simulink model "transition_RLSMC_2024aR1"  (R2024a)
settings: Solver=ode4  StartTime=0.0  StopTime=55  FixedStep=0.002  RelTol=1e-3
InitFcn:
  | model_init_param
values from neighbouring files (symbols this model uses):
  ModelInit_AngEuler = [ModelInit_phi, ModelInit_theta, ModelInit_psi]    [model_init_param.m]
  ModelInit_g = 9.80665    [model_init_param.m]
  ModelInit_PosE = [ModelInit_PosX, ModelInit_PosY, ModelInit_PosZ]    [model_init_param.m]
  ModelInit_RateB = [0, 0, 0]    [model_init_param.m]
  ModelInit_trim_da = 0    [model_init_param.m]
  ModelInit_trim_de = 0    [model_init_param.m]
  ModelInit_trim_dr = 0    [model_init_param.m]
  ModelInit_trim_dT = 0    [model_init_param.m]
  ModelInit_trim_u = ModelParam_mass/(4*ModelParam_rotor_Kf)    (= 0.533231666667)    [model_init_param.m]
  ModelInit_VelB = [ModelInit_Velx, ModelInit_Vely, ModelInit_Velz]    [model_init_param.m]
  ModelParam_Ixx = 2.957616474    [model_init_param.m]
  ModelParam_Iyy = 5.552907742    [model_init_param.m]
  ModelParam_Izz = 8.264706552    [model_init_param.m]
  ModelParam_mass = 31.9939    [model_init_param.m]
  ModelParam_rotor_Kf = 15    [model_init_param.m]
  ModelParam_rotor_Kt = 2.45    [model_init_param.m]
  ModelParam_rotor_x = 1.25    [model_init_param.m]
  ModelParam_rotor_y = 1.3    [model_init_param.m]
undefined symbols (not defined in the file or in its folder): Newton, Raphson, sigbuilder_block
libraries: aerolibconvert2 x5, aerolibasang x5, sharedutil x2, simulink x2, sharedtransform x2, aerolibatmos2 x1
settings Model: Creator=yifangfu  LastModifiedBy=yifangfu

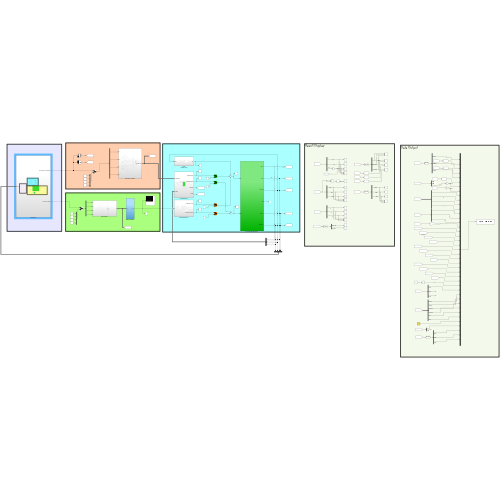
[thumbnail: Simulink's stored preview of the top-level diagram]
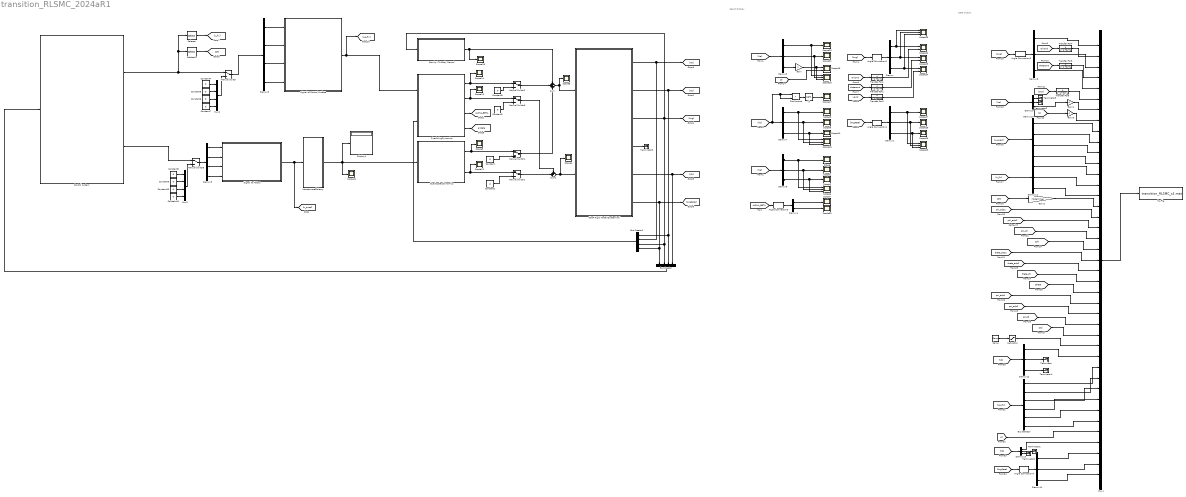
== system transition_RLSMC_2024aR1 ==
  note: Result Display
  note: Data Output
  6DoF Rigid Model(Quaternion) : Subsystem
  Actuator coefficiency : Subsystem
  Angle Conversion{1..5} (5 alike) : aerolibconvert2/Angle Conversion  IU=rad  OU=deg
  Bus Creator : BusCreator  Inputs=4
  Bus Creator1 : BusCreator  Inputs=4
  Bus Selector : BusSelector  OutputSignals=deup1,deup2,dedown1,dedown2,da1,da2
  Constant{,1..11} (12 alike) : Constant  Value=0
  Control system : Subsystem
  Demux{,1..2,6..9,11..14} (11 alike) : Demux  Outputs=3
  Demux10 : Demux
  Demux3 : Demux
  Demux4 : Demux  Outputs=2
  Demux5 : Demux
  Display4 : Display
  Dot Product : DotProduct  OutDataTypeStr=Inherit: Inherit via internal rule
  FixedWingDynamics : Subsystem
  Gain : Gain
  Gain1 : Gain  Gain=-1
  Gain2 : Gain  Gain=ModelInit_g
  Gain3 : Gain  Gain=-1
  Gravity (To Body Frame) : Subsystem
  Manual Switch{,1..2,4..6} (6 alike) : ManualSwitch
  Mux2 : Mux
  Mux3 : Mux
  Mux4 : Mux  Inputs=41
  QuadcoptersDynamics : Subsystem
  Ramp : simulink/Sources/Ramp  slope=0.65  start=0  InitialOutput=5
  Saturation : Saturate  UpperLimit=25
  Scope{,1..5,7..15,17,20..21,26..28,30} (22 alike) : Scope
  Scope{6,16,19,25,29} (5 alike) : Scope  NumInputPorts=3
  Scope{18,22..24} (4 alike) : Scope  NumInputPorts=2
  Selector : Selector  InputPortWidth=4  IndexOptions=Index vector (dialog)  Indices=[1 2 3]  OutputSizes=1
  Selector1 : Selector  InputPortWidth=4  IndexOptions=Index vector (dialog)  Indices=[4]  OutputSizes=1
  Signal to Control Surface : Subsystem
  Signal to Motors : Subsystem
  Sum : Sum  Inputs=+++
  Sum1 : Sum  Inputs=++|
  Terminator{,1..6} (7 alike) : Terminator
  To File : ToFile  Filename=transition_RLSMC_s1.mat  MatrixName=RLSMC_s1
  Transfer Fcn{1..6} (6 alike) : TransferFcn  Numerator=[4]  Denominator=[1 3 4]
  vt : Math  Operator=sqrt  SignedPower=on
  tag scope: ALPHA_BETA=global, airdata=global
  wires:
  Gain/1 -> Scope19/3, Scope18/1  "Height_m"
  Demux2/3 -> Gain/1  "Z_m"
  [yawd] -> Transfer Fcn3/1
  [Xe] -> Demux2/1
  Demux6/2 -> Scope6/2, Scope1/1  "vy"
  [ALPHA_BETA] -> Angle Conversion3/1
  [thetacmd] -> Transfer Fcn2/1
  Demux6/3 -> Scope6/3, Scope2/1  "vz"
  Demux7/3 -> Scope16/3, Scope10/1  "w(m/s)"
  Transfer Fcn3/1 -> Scope24/2
  Demux2/2 -> Scope19/2, Scope21/1  "Y_m"
  Dot Product/1 -> vt/1
  Demux2/1 -> Scope19/1, Scope20/1  "X_m"
  Demux/1 -> Scope22/1, Scope25/1  "phi(deg)"
  Demux4/1 -> Scope7/1  "alpha_deg"
  Demux/3 -> Scope24/1, Scope25/3  "psi(deg)"
  Demux1/3 -> Scope26/1, Scope29/3  "r(deg)"
  Demux1/1 -> Scope27/1, Scope29/1  "p(deg)"
  [Ve] -> Demux6/1
  [rollcmd] -> Transfer Fcn1/1
  Demux6/1 -> Scope6/1, Scope/1  "vx"
  Transfer Fcn2/1 -> Scope23/2
  [zd] -> Scope18/2
  [Ang] -> Angle Conversion2/1
  Angle Conversion1/1 -> Demux1/1
  Demux4/2 -> Scope30/1  "beta_deg"
  [Vb] -> Dot Product/2, Dot Product/1, Demux7/1
  Transfer Fcn1/1 -> Scope22/2
  [AngRate] -> Angle Conversion1/1
  Demux/2 -> Scope23/1, Scope25/2  "theta(deg)"
  Demux7/1 -> Scope16/1, Scope8/1  "u(m/s)"
  Angle Conversion3/1 -> Demux4/1
  vt/1 -> Scope17/1  "V(m/s)"
  Demux1/2 -> Scope28/1, Scope29/2  "q(deg)"
  Demux7/2 -> Scope16/2, Scope9/1  "v(m/s)"
  Angle Conversion2/1 -> Demux/1
  6DoF Rigid Model(Quaternion)/5("vb(m/s) ") -> [Vb], Bus Creator/4  "uvw"
  6DoF Rigid Model(Quaternion)/4(Rbe) -> Terminator3/1
  6DoF Rigid Model(Quaternion)/1(ve(m/s)) -> [Ve], Bus Creator1/2  "Ve"
  6DoF Rigid Model(Quaternion)/6("p,q,r(rad/s) ") -> Bus Creator1/4, Bus Creator/1, [AngRate]  "pqr"
  6DoF Rigid Model(Quaternion)/2("xe(m) ") -> [Xe], Bus Creator1/1, Bus Creator/3  "Xe"
  6DoF Rigid Model(Quaternion)/3(Euler(rad)) -> Gravity (To Body Frame)/1(Euler), [Ang], Bus Creator1/3, Bus Creator/2  "euler"
  Demux5/2 -> Signal to Motors/2(u2)
  Demux5/1 -> Signal to Motors/1(u1)
  Actuator coefficiency/1(u_out) -> QuadcoptersDynamics/1(u), Scope11/1, Display4/1
  Demux5/4 -> Signal to Motors/4(u4)
  Signal to Motors/1(u) -> [u_quad], Actuator coefficiency/1(u_in)
  Demux5/3 -> Signal to Motors/3(u3)
  Constant9/1 -> Mux3/2
  Constant10/1 -> Mux3/3
  Constant11/1 -> Mux3/4
  Mux3/1 -> Manual Switch5/2
  Constant8/1 -> Mux3/1
  Manual Switch5/1 -> Demux5/1
  Control system/2(ControlInputs_Rotors) -> Manual Switch5/1
  Bus Creator/1 -> Control system/1(Uav State)
  Sum/1 -> 6DoF Rigid Model(Quaternion)/1(fb), Scope3/1
  Gravity (To Body Frame)/1(g_b) -> Scope15/1, Sum/1
  FixedWingDynamics/3(alpha beta) -> [ALPHA_BETA]
  FixedWingDynamics/4(Airdata) -> [airdata]
  QuadcoptersDynamics/1(Quadcopters Force) -> Manual Switch4/1, Scope5/1
  FixedWingDynamics/1(FixedWing Force) -> Scope14/1, Manual Switch2/1
  Sum1/1 -> 6DoF Rigid Model(Quaternion)/2(Mb), Scope4/1
  QuadcoptersDynamics/2(Quadcopters Moment) -> Manual Switch1/1, Scope12/1
  FixedWingDynamics/2(FixedWing Moment) -> Manual Switch6/1, Scope13/1
  Constant/1 -> Manual Switch4/2
  Constant1/1 -> Manual Switch1/2
  Manual Switch1/1 -> Sum1/2
  Manual Switch4/1 -> Sum/3
  Constant2/1 -> Manual Switch6/2
  Manual Switch6/1 -> Sum1/1
  Manual Switch2/1 -> Sum/2
  Constant3/1 -> Manual Switch2/2
  Bus Creator1/1 -> FixedWingDynamics/2(UavState)
  Signal to Control Surface/1(ControlSurface) -> [ua_fix], FixedWingDynamics/1(ControlSurface)
  Constant4/1 -> Mux2/1
  Constant7/1 -> Mux2/4
  Mux2/1 -> Manual Switch/2
  Constant5/1 -> Mux2/2
  Manual Switch/1 -> Demux3/1
  Constant6/1 -> Mux2/3
  Demux3/1 -> Signal to Control Surface/1(de)
  Demux3/2 -> Signal to Control Surface/2(da)
  Demux3/3 -> Signal to Control Surface/3(dr)
  Demux3/4 -> Signal to Control Surface/4(dT)
  Control system/1(ControlInputs_ControlSurfaces) -> Selector1/1, Selector/1, Manual Switch/1
  [stheta] -> Mux4/24
  Demux11/2 -> Mux4/14  "de"
  [phi_adp2] -> Mux4/18
  Demux12/1 -> Mux4/30  "u(m/s)"
  [zd] -> Gain3/1
  [phi_adp1] -> Mux4/17
  Demux10/3 -> Mux4/11  "u3"
  Demux11/1 -> Mux4/13  "da"
  Gain2/1 -> Mux4/16
  [Xe] -> Demux9/1
  Transfer Fcn4/1 -> Mux4/2
  [dT] -> Gain2/1
  Demux9/2 -> Terminator6/1  "Y_m"
  Demux9/3 -> Gain1/1  "Z_m"
  Ramp/1 -> Saturation/1
  Transfer Fcn6/1 -> Mux4/6
  Demux8/3 -> Mux4/5  "psi(deg)"
  [Ang] -> Angle Conversion5/1
  Demux8/2 -> Mux4/3  "theta(deg)"
  Angle Conversion5/1 -> Demux8/1
  [rollcmd] -> Transfer Fcn4/1
  Gain1/1 -> Mux4/7  "Height_m"
  Demux12/3 -> Terminator4/1  "w(m/s)"
  Demux12/2 -> Terminator/1  "v(m/s)"
  [spsi] -> Mux4/28
  [psi_adp1] -> Mux4/25
  [psi_adp2] -> Mux4/26
  Demux9/1 -> Terminator5/1  "X_m"
  [phi_k3] -> Mux4/19
  Demux10/2 -> Mux4/10  "u2"
  [Vb] -> Demux12/1
  Saturation/1 -> Mux4/29  "ud"
  Demux10/4 -> Mux4/12  "u4"
  Demux10/1 -> Mux4/9  "u1"
  [psi_k3] -> Mux4/27
  Transfer Fcn5/1 -> Mux4/4
  Demux11/3 -> Mux4/15  "dr"
  [u_quad] -> Demux10/1
  Demux8/1 -> Mux4/1  "phi(deg)"
  [u_fix] -> Demux11/1
  [theta_adp2] -> Mux4/22
  [theta_k3] -> Mux4/23
  [yawd] -> Transfer Fcn6/1
  [theta_adp1] -> Mux4/21
  [thetacmd] -> Transfer Fcn5/1
  [sphi] -> Mux4/20
  Selector/1 -> [u_fix]
  Selector1/1 -> [dT]
  Mux4/1 -> To File/1
  Gain3/1 -> Mux4/8  "Height_m"
  Bus Selector/2 -> Mux4/32  "<deup2>"
  Bus Selector/1 -> Mux4/31  "<deup1>"
  Bus Selector/6 -> Mux4/36  "<da2>"
  Bus Selector/5 -> Mux4/35  "<da1>"
  Bus Selector/4 -> Mux4/34  "<dedown2>"
  Bus Selector/3 -> Mux4/33  "<dedown1>"
  [ua_fix] -> Bus Selector/1
  Demux13/1 -> Mux4/38
  Demux13/3 -> Terminator2/1
  [ud] -> Mux4/37
  [Vb] -> Demux13/1
  Demux13/2 -> Terminator1/1
  Angle Conversion4/1 -> Demux14/1
  [AngRate] -> Angle Conversion4/1
  Demux14/1 -> Mux4/39  "p(deg)"
  Demux14/2 -> Mux4/40  "q(deg)"
  Demux14/3 -> Mux4/41  "r(deg)"

== system transition_RLSMC_2024aR1/6DoF Rigid Model(Quaternion) ==
  fb : Inport
  Mb : Inport  Port=2
  Rigid-Body Dynamic Model : Subsystem
  "Rigid-Body Kinematic Model " : Subsystem
  ve(m/s) : Outport  VectorParamsAs1DForOutWhenUnconnected=off
  "xe(m) " : Outport  Port=2  VectorParamsAs1DForOutWhenUnconnected=off
  Euler(rad) : Outport  Port=3  VectorParamsAs1DForOutWhenUnconnected=off
  Rbe : Outport  Port=4  VectorParamsAs1DForOutWhenUnconnected=off
  "vb(m/s) " : Outport  Port=5  VectorParamsAs1DForOutWhenUnconnected=off
  "p,q,r(rad/s) " : Outport  Port=6  VectorParamsAs1DForOutWhenUnconnected=off
  wires:
  Rigid-Body Dynamic Model/1("p,q,r ") -> "p,q,r(rad/s) "/1, "Rigid-Body Kinematic Model "/1(pqr)
  "Rigid-Body Kinematic Model "/1(Euler) -> Euler(rad)/1
  "Rigid-Body Kinematic Model "/3(Rbe) -> Rbe/1, Rigid-Body Dynamic Model/3(Rbe)
  Mb/1 -> Rigid-Body Dynamic Model/1(Mb)
  fb/1 -> Rigid-Body Dynamic Model/2(f)
  Rigid-Body Dynamic Model/2(ve) -> ve(m/s)/1, "Rigid-Body Kinematic Model "/2(ve)
  Rigid-Body Dynamic Model/3("vb ") -> "vb(m/s) "/1
  "Rigid-Body Kinematic Model "/2("xe ") -> "xe(m) "/1

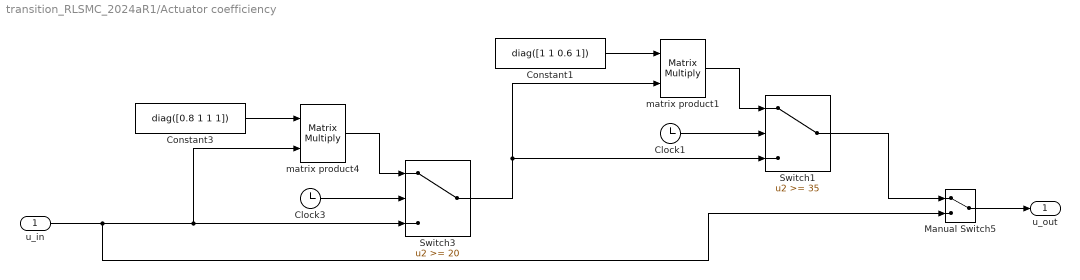
== system transition_RLSMC_2024aR1/Actuator coefficiency ==
  u_in : Inport
  Clock1 : Clock
  Clock3 : Clock
  Constant1 : Constant  Value=diag([1 1 0.6 1])
  Constant3 : Constant  Value=diag([0.8 1 1 1])
  Manual Switch5 : ManualSwitch
  Switch1 : Switch  Threshold=35  SaturateOnIntegerOverflow=off  InputSameDT=off
  Switch3 : Switch  Threshold=20  SaturateOnIntegerOverflow=off  InputSameDT=off
  matrix product1 : Product  Multiplication=Matrix(*)
  matrix product4 : Product  Multiplication=Matrix(*)
  u_out : Outport
  wires:
  Constant3/1 -> matrix product4/1
  Clock3/1 -> Switch3/2
  matrix product4/1 -> Switch3/1
  u_in/1 -> Switch3/3, matrix product4/2, Manual Switch5/2
  Manual Switch5/1 -> u_out/1
  matrix product1/1 -> Switch1/1
  Switch3/1 -> matrix product1/2, Switch1/3
  Clock1/1 -> Switch1/2
  Constant1/1 -> matrix product1/1
  Switch1/1 -> Manual Switch5/1

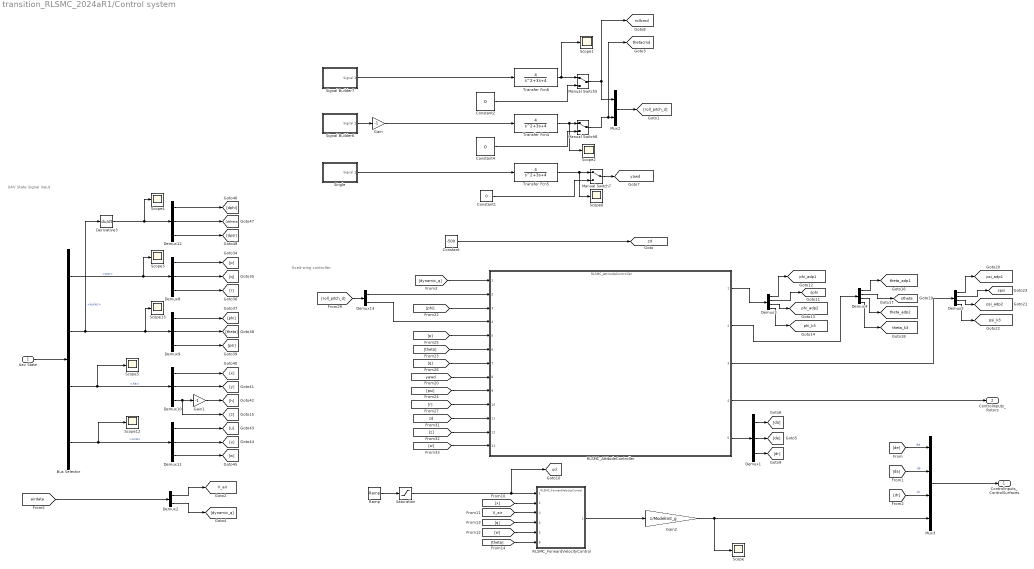
== system transition_RLSMC_2024aR1/Control system ==
  note: UAV State Signal Input
  note: fixed-wing controller
  Uav State : Inport
  Bus Selector : BusSelector  OutputSignals=pqr,euler,Xe,uvw
  Constant : Constant  Value=-500
  Constant1 : Constant  Value=0
  Constant2 : Constant  Value=0
  Constant4 : Constant  Value=0
  Demux{1,8..12} (6 alike) : Demux  Outputs=3
  Demux13 : Demux  Outputs=2
  Demux2 : Demux  Outputs=2
  Demux3 : Demux
  Demux4 : Demux
  Demux5 : Demux
  Derivative3 : Derivative
  Gain : Gain  Gain=-1
  Gain1 : Gain  Gain=-1
  Gain2 : Gain  Gain=1/ModelInit_g
  Manual Switch5 : ManualSwitch
  Manual Switch7 : ManualSwitch
  Manual Switch8 : ManualSwitch
  Mux2 : Mux  Inputs=2
  Mux3 : Mux
  RLSMC_AttitudeController : ModelReference  ModelNameDialog=RLSMC_AttitudeController  ModelReferenceVersion=2.2  CopyOfModelProtected=on
  RLSMC_ForwardVelocityControl : ModelReference  ModelNameDialog=RLSMC_ForwardVelocityControl  ModelReferenceVersion=2.1  CopyOfModelProtected=on
  Ramp : simulink/Sources/Ramp  slope=0.25  start=0  InitialOutput=5
  Saturation : Saturate  UpperLimit=16
  Scope{,1..6,12..13} (9 alike) : Scope
  Signal Builder6 : Subsystem  Tag=STV Subsys  LoadFcn=sigbuilder_block('load');  StartFcn=sigbuilder_block('start');  StopFcn=sigbuilder_block('stop');  ClipboardFcn=sigbuilder_block('clipboard');  mask(Sigbuilder block){tuvar=[0:10]}
      mask help: Simulink:masks:SigbuilderBlock_MD
      mask init:
      | if ~strcmp(get_param(bdroot(gcbh),'SimulationStatus'),'stopped') tuvar = sigbuilder_block('maskInit'); end
      settings: CopyFcn=sigbuilder_block('copy');  DeleteFcn=sigbuilder_block('delete');  ModelCloseFcn=sigbuilder_block('modelClose');  PreSaveFcn=sigbuilder_block('preSave');  PauseFcn=sigbuilder_block('pause');  ContinueFcn=sigbuilder_block('continue');  NameChangeFcn=sigbuilder_block('namechange');  OpenFcn=sigbuilder_block('open',[5.5 42 1109 536 ]);  CloseFcn=sigbuilder_block('close');
      mask Display: plot(0, 0, 100, 100,[2, 2, 32, 32, 2], [68, 8, 8, 68, 68],[32, 2], [38, 38], [32, 19, 2],[53, 60, 44], [32, 17, 17, 2],[16, 16, 31, 31]);txt = getActiveGroup(gcbh);text(2, 100, txt,'verticalAlignment', 'top');
  Signal Builder7 : Subsystem  Tag=STV Subsys  LoadFcn=sigbuilder_block('load');  StartFcn=sigbuilder_block('start');  StopFcn=sigbuilder_block('stop');  ClipboardFcn=sigbuilder_block('clipboard');  mask(Sigbuilder block){tuvar=[0:10]}
      mask help: Simulink:masks:SigbuilderBlock_MD
      mask init:
      | if ~strcmp(get_param(bdroot(gcbh),'SimulationStatus'),'stopped') tuvar = sigbuilder_block('maskInit'); end
      settings: CopyFcn=sigbuilder_block('copy');  DeleteFcn=sigbuilder_block('delete');  ModelCloseFcn=sigbuilder_block('modelClose');  PreSaveFcn=sigbuilder_block('preSave');  PauseFcn=sigbuilder_block('pause');  ContinueFcn=sigbuilder_block('continue');  NameChangeFcn=sigbuilder_block('namechange');  OpenFcn=sigbuilder_block('open',[498.5 117 550.5 400.5 ]);  CloseFcn=sigbuilder_block('close');
      mask Display: plot(0, 0, 100, 100,[2, 2, 32, 32, 2], [68, 8, 8, 68, 68],[32, 2], [38, 38], [32, 19, 2],[53, 60, 44], [32, 17, 17, 2],[16, 16, 31, 31]);txt = getActiveGroup(gcbh);text(2, 100, txt,'verticalAlignment', 'top');
  Single : Subsystem  Tag=STV Subsys  LoadFcn=sigbuilder_block('load');  StartFcn=sigbuilder_block('start');  StopFcn=sigbuilder_block('stop');  ClipboardFcn=sigbuilder_block('clipboard');  mask(Sigbuilder block){tuvar=[0:10]}
      mask help: Simulink:masks:SigbuilderBlock_MD
      mask init:
      | if ~strcmp(get_param(bdroot(gcbh),'SimulationStatus'),'stopped') tuvar = sigbuilder_block('maskInit'); end
      settings: CopyFcn=sigbuilder_block('copy');  DeleteFcn=sigbuilder_block('delete');  ModelCloseFcn=sigbuilder_block('modelClose');  PreSaveFcn=sigbuilder_block('preSave');  PauseFcn=sigbuilder_block('pause');  ContinueFcn=sigbuilder_block('continue');  NameChangeFcn=sigbuilder_block('namechange');  OpenFcn=sigbuilder_block('open',[5.5 42 1109 536 ]);  CloseFcn=sigbuilder_block('close');
      mask Display: plot(0, 0, 100, 100,[2, 2, 32, 32, 2], [68, 8, 8, 68, 68],[32, 2], [38, 38], [32, 19, 2],[53, 60, 44], [32, 17, 17, 2],[16, 16, 31, 31]);txt = getActiveGroup(gcbh);text(2, 100, txt,'verticalAlignment', 'top');
  Transfer Fcn4 : TransferFcn  Numerator=[4]  Denominator=[1 3 4]
  Transfer Fcn5 : TransferFcn  Numerator=[4]  Denominator=[1 3 4]
  Transfer Fcn6 : TransferFcn  Numerator=[4]  Denominator=[1 3 4]
  ControlInputs_ControlSurfaces : Outport
  ControlInputs_Rotors : Outport  Port=2
  tag scope: V_air=global, phi_adp1=global, phi_adp2=global, phi_k3=global, psi_adp1=global, psi_adp2=global, psi_k3=global, rollcmd=global, sphi=global, spsi=global, stheta=global, theta_adp1=global, theta_adp2=global, theta_k3=global, thetacmd=global, ud=global, yawd=global, zd=global
  wires:
  Demux8/2 -> [q]
  Demux9/3 -> [psi]
  Demux11/2 -> [v]
  Gain1/1 -> [h]
  Demux12/3 -> [dpsi]
  Uav State/1 -> Bus Selector/1
  Demux11/3 -> [w]
  Demux12/2 -> [dtheta]
  Demux12/1 -> [dphi]
  Demux10/1 -> [x]
  Demux9/2 -> [theta]
  Demux8/1 -> [p]
  Demux10/2 -> [y]
  Demux9/1 -> [phi]
  Derivative3/1 -> Scope4/1, Demux12/1
  [roll_pitch_d] -> Demux13/1
  Demux8/3 -> [r]
  Bus Selector/4 -> Demux11/1, Scope12/1  "<uvw>"
  Bus Selector/1 -> Scope3/1, Demux8/1  "<pqr>"
  Demux10/3 -> [z], Gain1/1
  Demux11/1 -> [u]
  Bus Selector/3 -> Demux10/1, Scope5/1  "<Xe>"
  Bus Selector/2 -> Scope13/1, Demux9/1, Derivative3/1  "<euler>"
  Constant1/1 -> Manual Switch7/2
  Manual Switch5/1 -> [rollcmd], Mux2/1
  Signal Builder6/1(Signal 1) -> Gain/1
  Manual Switch7/1 -> [yawd]
  Manual Switch8/1 -> [thetacmd], Mux2/2
  Constant4/1 -> Manual Switch8/2
  Constant2/1 -> Manual Switch5/2
  Transfer Fcn5/1 -> Scope6/1, Manual Switch7/1
  Transfer Fcn4/1 -> Scope2/1, Manual Switch8/1
  Transfer Fcn6/1 -> Scope1/1, Manual Switch5/1
  Mux2/1 -> [roll_pitch_d]
  Constant/1 -> [zd]
  Demux2/1 -> [V_air]
  [airdata] -> Demux2/1
  Demux2/2 -> [dynamic_q]
  [theta] -> RLSMC_ForwardVelocityControl/6
  [q] -> RLSMC_ForwardVelocityControl/4
  Ramp/1 -> Saturation/1
  Saturation/1 -> [ud], RLSMC_ForwardVelocityControl/1
  [w] -> RLSMC_ForwardVelocityControl/5
  [V_air] -> RLSMC_ForwardVelocityControl/3
  [x] -> RLSMC_ForwardVelocityControl/2
  Demux1/3 -> [dr]
  Demux1/2 -> [de]
  Demux1/1 -> [da]
  [dr] -> Mux3/3  "dr"
  [da] -> Mux3/2  "da"
  [de] -> Mux3/1  "de"
  Gain2/1 -> Scope/1, Mux3/4
  Mux3/1 -> ControlInputs_ControlSurfaces/1
  Single/1(Signal 1) -> Transfer Fcn5/1
  RLSMC_ForwardVelocityControl/1 -> Gain2/1
  Demux3/1 -> [phi_adp1]
  Demux3/2 -> [sphi]
  Demux3/3 -> [phi_adp2]
  Demux3/4 -> [phi_k3]
  Demux4/1 -> [theta_adp1]
  Demux4/2 -> [stheta]
  Demux4/3 -> [theta_adp2]
  Demux4/4 -> [theta_k3]
  Demux5/1 -> [psi_adp1]
  Demux5/2 -> [spsi]
  Demux5/3 -> [psi_adp2]
  Demux5/4 -> [psi_k3]
  [dynamic_q] -> RLSMC_AttitudeController/1
  Demux13/1 -> RLSMC_AttitudeController/2
  [phi] -> RLSMC_AttitudeController/3
  Demux13/2 -> RLSMC_AttitudeController/4
  [p] -> RLSMC_AttitudeController/5
  [theta] -> RLSMC_AttitudeController/6
  [q] -> RLSMC_AttitudeController/7
  [yawd] -> RLSMC_AttitudeController/8
  [psi] -> RLSMC_AttitudeController/9
  [r] -> RLSMC_AttitudeController/10
  [zd] -> RLSMC_AttitudeController/11
  [z] -> RLSMC_AttitudeController/12
  [w] -> RLSMC_AttitudeController/13
  RLSMC_AttitudeController/1 -> Demux3/1
  RLSMC_AttitudeController/4 -> ControlInputs_Rotors/1
  RLSMC_AttitudeController/2 -> Demux4/1
  RLSMC_AttitudeController/5 -> Demux1/1
  RLSMC_AttitudeController/3 -> Demux5/1
  Gain/1 -> Transfer Fcn4/1
  Signal Builder7/1(Signal 1) -> Transfer Fcn6/1

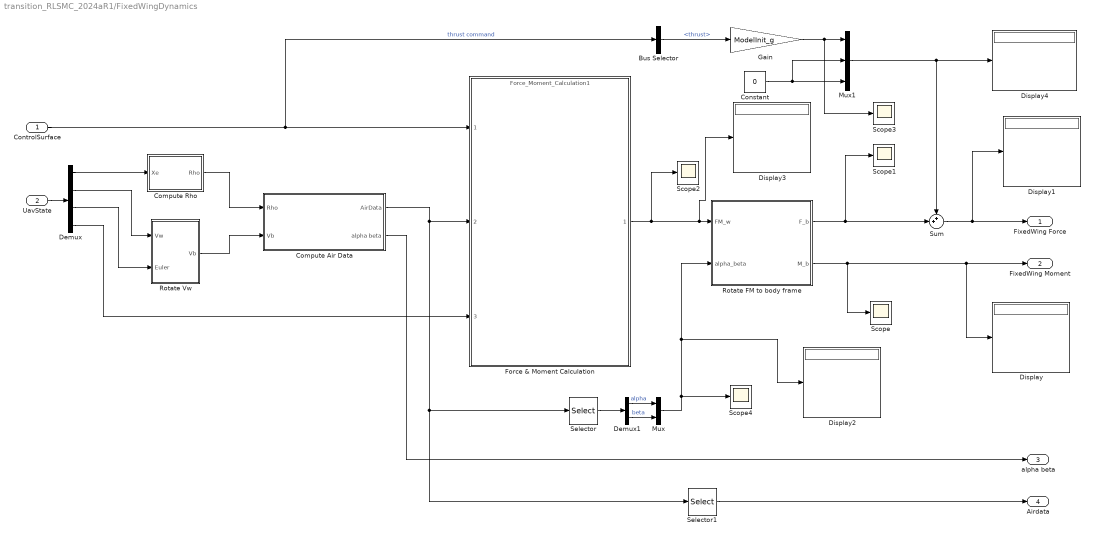
== system transition_RLSMC_2024aR1/FixedWingDynamics ==
  ControlSurface : Inport
  UavState : Inport  Port=2
  Bus Selector : BusSelector  OutputSignals=thrust
  Compute Air Data : Subsystem  TreatAsAtomicUnit=on  VariantControl=use_aerospace_blocks == 1
  Compute Rho : Subsystem
  Constant : Constant  Value=0
  Demux : Demux
  Demux1 : Demux  Outputs=2
  Display{,1..4} (5 alike) : Display
  Force & Moment Calculation : ModelReference  ModelNameDialog=Force_Moment_Calculation1  ModelReferenceVersion=2.1  CopyOfModelProtected=on
  Gain : Gain  Gain=ModelInit_g
  Mux : Mux  Inputs=2
  Mux1 : Mux  Inputs=3
  Rotate FM to body frame : Subsystem
  Rotate Vw : Subsystem
  Scope{,1..4} (5 alike) : Scope
  Selector : Selector  InputPortWidth=4  IndexOptions=Index vector (dialog)  Indices=[ 1 2]  OutputSizes=1
  Selector1 : Selector  InputPortWidth=4  IndexOptions=Index vector (dialog)  Indices=[ 3 4]  OutputSizes=1
  Sum : Sum  Inputs=++|
  FixedWing Force : Outport
  FixedWing Moment : Outport  Port=2
  alpha beta : Outport  Port=3
  Airdata : Outport  Port=4
  wires:
  Demux/1 -> Compute Rho/1(Xe)
  Demux/3 -> Rotate Vw/2(Euler)
  Rotate Vw/1(Vb) -> Compute Air Data/2(Vb)
  Demux/2 -> Rotate Vw/1(Vw)
  Compute Rho/1(Rho) -> Compute Air Data/1(Rho)
  UavState/1 -> Demux/1
  ControlSurface/1 -> Force & Moment Calculation/1, Bus Selector/1  "thrust command"
  Demux/4 -> Force & Moment Calculation/3
  Mux/1 -> Rotate FM to body frame/2(alpha_beta), Display2/1, Scope4/1
  Rotate FM to body frame/2(M_b) -> Scope/1, Display/1, FixedWing Moment/1
  Force & Moment Calculation/1 -> Scope2/1, Display3/1, Rotate FM to body frame/1(FM_w)
  Compute Air Data/1(AirData) -> Force & Moment Calculation/2, Selector1/1, Selector/1
  Demux1/1 -> Mux/1  "alpha"
  Demux1/2 -> Mux/2  "beta"
  Selector/1 -> Demux1/1
  Rotate FM to body frame/1(F_b) -> Scope1/1, Sum/2
  Sum/1 -> Display1/1, FixedWing Force/1
  Constant/1 -> Mux1/2, Mux1/3
  Mux1/1 -> Display4/1, Sum/1
  Gain/1 -> Scope3/1, Mux1/1
  Bus Selector/1 -> Gain/1  "<thrust>"
  Compute Air Data/2(alpha beta) -> alpha beta/1
  Selector1/1 -> Airdata/1

== system transition_RLSMC_2024aR1/Gravity (To Body Frame) ==
  Euler : Inport
  Gravitational Force : Constant  Value=[0 0 ModelParam_mass*ModelInit_g]  VectorParams1D=off
      settings: AttributesFormatString=%<Value>
  Rotate g to Body Frame : Subsystem
  Signal Specification : SignalSpecification  Unit=kg*m/s^2
  g_b : Outport
  wires:
  Gravitational Force/1 -> Signal Specification/1
  Rotate g to Body Frame/1(g_b) -> g_b/1
  Signal Specification/1 -> Rotate g to Body Frame/2(Gravity Force)
  Euler/1 -> Rotate g to Body Frame/1(Euler)

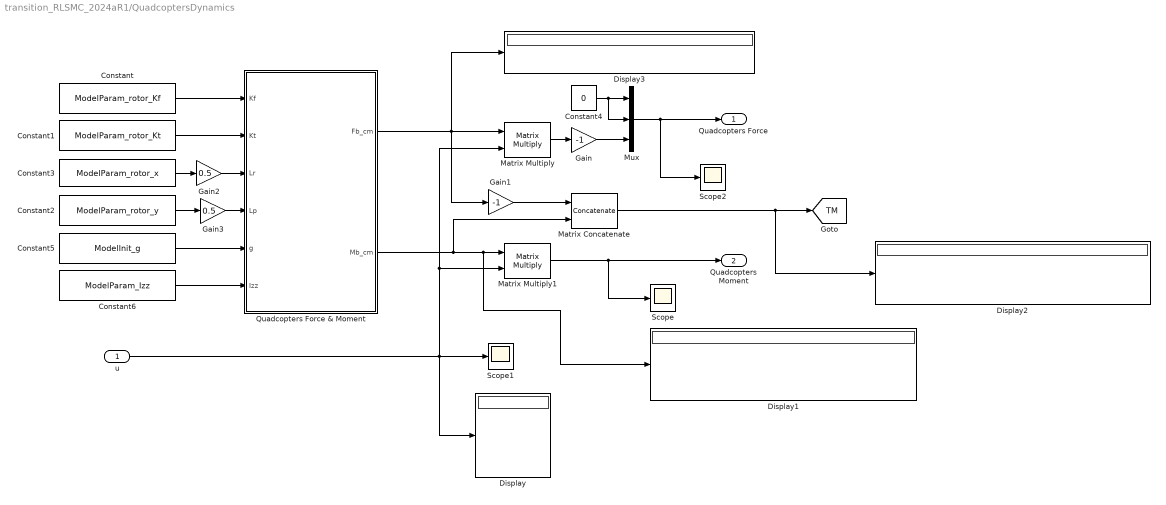
== system transition_RLSMC_2024aR1/QuadcoptersDynamics ==
  u : Inport
  Constant : Constant  Value=ModelParam_rotor_Kf
  Constant1 : Constant  Value=ModelParam_rotor_Kt
  Constant2 : Constant  Value=ModelParam_rotor_y
  Constant3 : Constant  Value=ModelParam_rotor_x
  Constant4 : Constant  Value=0
  Constant5 : Constant  Value=ModelInit_g
  Constant6 : Constant  Value=ModelParam_Izz
  Display{,1..3} (4 alike) : Display
  Gain : Gain  Gain=-1
  Gain1 : Gain  Gain=-1
  Gain2 : Gain  Gain=0.5
  Gain3 : Gain  Gain=0.5
  Matrix Concatenate : Concatenate  Mode=Multidimensional array
  Matrix Multiply : Product  Multiplication=Matrix(*)
  Matrix Multiply1 : Product  Multiplication=Matrix(*)
  Mux : Mux  Inputs=3
  Quadcopters Force & Moment : MATLAB Function  TreatAsAtomicUnit=on
  Scope : Scope
  Scope1 : Scope
  Scope2 : Scope
  Quadcopters Force : Outport
  Quadcopters Moment : Outport  Port=2
  tag scope: TM=global
  wires:
  Constant/1 -> Quadcopters Force & Moment/1(Kf)
  Constant1/1 -> Quadcopters Force & Moment/2(Kt)
  Constant3/1 -> Gain2/1
  Quadcopters Force & Moment/1(Fb_cm) -> Gain1/1, Display3/1, Matrix Multiply/1
  Quadcopters Force & Moment/2(Mb_cm) -> Matrix Concatenate/2, Display1/1, Matrix Multiply1/1
  u/1 -> Display/1, Matrix Multiply/2, Matrix Multiply1/2, Scope1/1
  Matrix Multiply/1 -> Gain/1
  Gain/1 -> Mux/3
  Constant4/1 -> Mux/2, Mux/1
  Mux/1 -> Scope2/1, Quadcopters Force/1
  Matrix Multiply1/1 -> Scope/1, Quadcopters Moment/1
  Constant2/1 -> Gain3/1
  Constant5/1 -> Quadcopters Force & Moment/5(g)
  Constant6/1 -> Quadcopters Force & Moment/6(Izz)
  Matrix Concatenate/1 -> Display2/1, [TM]
  Gain1/1 -> Matrix Concatenate/1
  Gain2/1 -> Quadcopters Force & Moment/3(Lr)
  Gain3/1 -> Quadcopters Force & Moment/4(Lp)

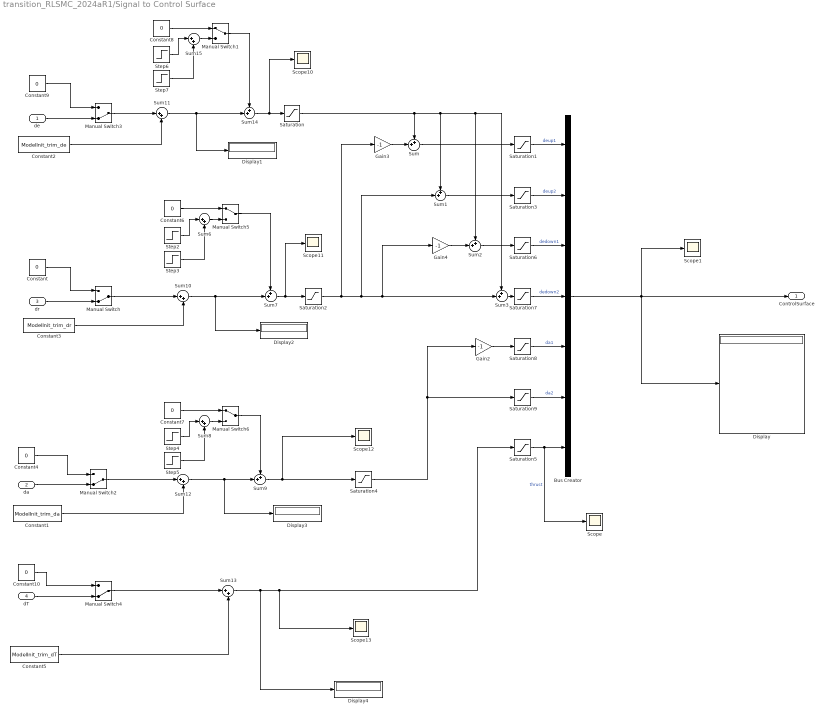
== system transition_RLSMC_2024aR1/Signal to Control Surface ==
  de : Inport
  da : Inport  Port=2
  dr : Inport  Port=3
  dT : Inport  Port=4
  Bus Creator : BusCreator  Inputs=7
  Constant{,4,6..10} (7 alike) : Constant  Value=0
  Constant1 : Constant  Value=ModelInit_trim_da
  Constant2 : Constant  Value=ModelInit_trim_de
  Constant3 : Constant  Value=ModelInit_trim_dr
  Constant5 : Constant  Value=ModelInit_trim_dT
  Display{,1..4} (5 alike) : Display
  Gain2 : Gain  Gain=-1
  Gain3 : Gain  Gain=-1
  Gain4 : Gain  Gain=-1
  Manual Switch{,2..4} (4 alike) : ManualSwitch  CurrentSetting=0
  Manual Switch1 : ManualSwitch
  Manual Switch5 : ManualSwitch
  Manual Switch6 : ManualSwitch
  Saturation{,1..4,6..7} (7 alike) : Saturate  UpperLimit=25  LowerLimit=-25
  Saturation5 : Saturate  UpperLimit=12  LowerLimit=-12  ZeroCross=off
  Saturation8 : Saturate  UpperLimit=20  LowerLimit=-20
  Saturation9 : Saturate  UpperLimit=20  LowerLimit=-20
  Scope{,1,10..13} (6 alike) : Scope
  Step2 : Step  Time=2  SampleTime=0
  Step3 : Step  Time=2.1  After=-1  SampleTime=0
  Step4 : Step  Time=2  SampleTime=0
  Step5 : Step  Time=2.5  After=-1  SampleTime=0
  Step6 : Step  Time=2  After=0.5  SampleTime=0
  Step7 : Step  Time=2.1  After=-0.5  SampleTime=0
  Sum{,1..3,7,9,14} (7 alike) : Sum  Inputs=++|
  Sum{6,8,10..13,15} (7 alike) : Sum  Inputs=|++
  ControlSurface : Outport
  wires:
  Saturation/1 -> Sum3/1, Sum2/1, Sum1/1, Sum/1
  Gain3/1 -> Sum/2
  Sum6/1 -> Manual Switch5/2
  Step3/1 -> Sum6/2
  Saturation4/1 -> Gain2/1, Saturation9/1
  Sum7/1 -> Saturation2/1, Scope11/1
  Constant5/1 -> Sum13/2
  Step5/1 -> Sum8/2
  Sum/1 -> Saturation1/1
  Step4/1 -> Sum8/1
  Saturation2/1 -> Sum3/2, Gain4/1, Sum1/2, Gain3/1
  Constant2/1 -> Sum11/2
  Sum13/1 -> Display4/1, Saturation5/1, Scope13/1
  Sum1/1 -> Saturation3/1
  Step2/1 -> Sum6/1
  Constant6/1 -> Manual Switch5/1
  Constant1/1 -> Sum12/2
  Step7/1 -> Sum15/2
  Sum2/1 -> Saturation6/1
  Constant7/1 -> Manual Switch6/1
  Constant8/1 -> Manual Switch1/1
  Manual Switch6/1 -> Sum9/1
  Manual Switch5/1 -> Sum7/1
  Gain2/1 -> Saturation8/1
  Sum3/1 -> Saturation7/1
  Sum8/1 -> Manual Switch6/2
  Sum14/1 -> Scope10/1, Saturation/1
  Gain4/1 -> Sum2/2
  Sum9/1 -> Scope12/1, Saturation4/1
  Saturation5/1 -> Scope/1, Bus Creator/7  "thrust"
  Sum10/1 -> Display2/1, Sum7/2
  Sum12/1 -> Display3/1, Sum9/2
  Constant3/1 -> Sum10/2
  Sum15/1 -> Manual Switch1/2
  Step6/1 -> Sum15/1
  Sum11/1 -> Display1/1, Sum14/2
  Manual Switch1/1 -> Sum14/1
  Bus Creator/1 -> Scope1/1, ControlSurface/1, Display/1
  Saturation1/1 -> Bus Creator/1  "deup1"
  Saturation3/1 -> Bus Creator/2  "deup2"
  Saturation6/1 -> Bus Creator/3  "dedown1"
  Saturation7/1 -> Bus Creator/4  "dedown2"
  Saturation8/1 -> Bus Creator/5  "da1"
  Saturation9/1 -> Bus Creator/6  "da2"
  Manual Switch/1 -> Sum10/1
  dr/1 -> Manual Switch/2
  Constant/1 -> Manual Switch/1
  Constant4/1 -> Manual Switch2/1
  Manual Switch2/1 -> Sum12/1
  da/1 -> Manual Switch2/2
  Constant9/1 -> Manual Switch3/1
  Manual Switch3/1 -> Sum11/1
  de/1 -> Manual Switch3/2
  Manual Switch4/1 -> Sum13/1
  dT/1 -> Manual Switch4/2
  Constant10/1 -> Manual Switch4/1

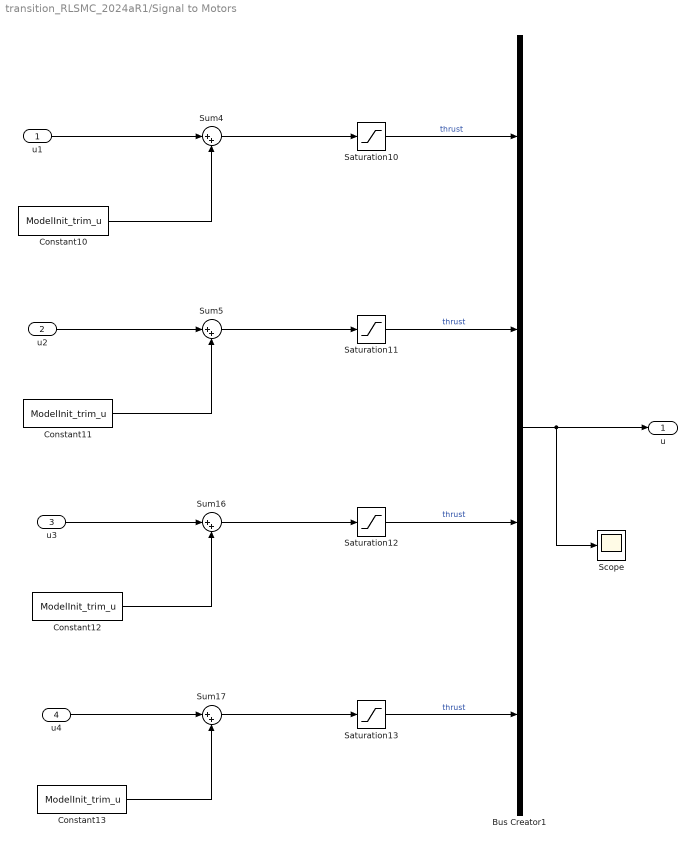
== system transition_RLSMC_2024aR1/Signal to Motors ==
  u1 : Inport
  u2 : Inport  Port=2
  u3 : Inport  Port=3
  u4 : Inport  Port=4
  Bus Creator1 : BusCreator  Inputs=4
  Constant{10..13} (4 alike) : Constant  Value=ModelInit_trim_u
  Saturation{10..13} (4 alike) : Saturate  UpperLimit=1  LowerLimit=0
  Scope : Scope
  Sum{4..5,16..17} (4 alike) : Sum  Inputs=|++
  u : Outport
  wires:
  u1/1 -> Sum4/1
  Constant10/1 -> Sum4/2
  u2/1 -> Sum5/1
  Constant11/1 -> Sum5/2
  u3/1 -> Sum16/1
  Constant12/1 -> Sum16/2
  u4/1 -> Sum17/1
  Constant13/1 -> Sum17/2
  Sum4/1 -> Saturation10/1
  Sum5/1 -> Saturation11/1
  Sum16/1 -> Saturation12/1
  Sum17/1 -> Saturation13/1
  Saturation10/1 -> Bus Creator1/1  "thrust"
  Saturation11/1 -> Bus Creator1/2  "thrust"
  Saturation12/1 -> Bus Creator1/3  "thrust"
  Saturation13/1 -> Bus Creator1/4  "thrust"
  Bus Creator1/1 -> Scope/1, u/1

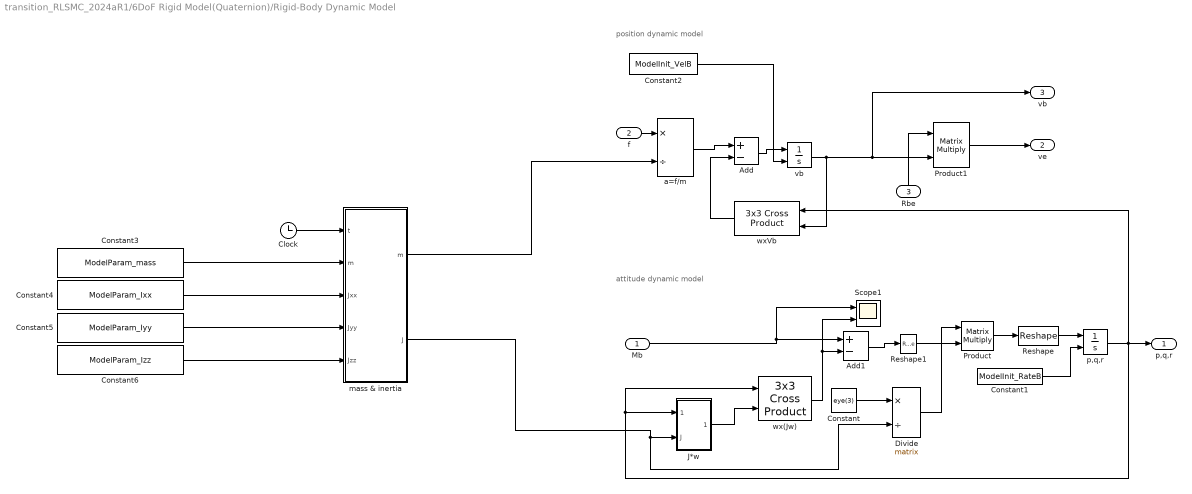
== system transition_RLSMC_2024aR1/6DoF Rigid Model(Quaternion)/Rigid-Body Dynamic Model ==
  note: attitude dynamic model
  note: position dynamic model
  Mb : Inport
  f : Inport  Port=2
  Rbe : Inport  Port=3
  Add : Sum  Inputs=+-
  Add1 : Sum  Inputs=+-
  Clock : Clock
  Constant : Constant  Value=eye(3)
  Constant1 : Constant  Value=ModelInit_RateB
  Constant2 : Constant  Value=ModelInit_VelB
  Constant3 : Constant  Value=ModelParam_mass
  Constant4 : Constant  Value=ModelParam_Ixx
  Constant5 : Constant  Value=ModelParam_Iyy
  Constant6 : Constant  Value=ModelParam_Izz
  Divide : Product  Inputs=*/  Multiplication=Matrix(*)
  J*w : Subsystem
  Product : Product  Multiplication=Matrix(*)
  Product1 : Product  Multiplication=Matrix(*)
  Reshape : Reshape  OutputDimensionality=Customize  OutputDimensions=[3,1]
  Reshape1 : Reshape  OutputDimensionality=Column vector (2-D)
  Scope1 : Scope  NumInputPorts=2
  a=f/m : Product  Inputs=*/
  mass & inertia : MATLAB Function  TreatAsAtomicUnit=on
  p,q,r : Integrator  InitialConditionSource=external
  vb : Integrator  InitialConditionSource=external
  wx(Jw) : sharedutil/3x3 Cross Product  aMode=aMode
  wxVb : sharedutil/3x3 Cross Product  aMode=aMode
  "p,q,r " : Outport  VectorParamsAs1DForOutWhenUnconnected=off
  ve : Outport  Port=2  VectorParamsAs1DForOutWhenUnconnected=off
  "vb " : Outport  Port=3  VectorParamsAs1DForOutWhenUnconnected=off
  wires:
  Product/1 -> Reshape/1
  Reshape1/1 -> Product/2
  Constant/1 -> Divide/1
  Divide/1 -> Product/1
  Add1/1 -> Reshape1/1
  mass & inertia/2(J) -> J*w/2(J), Divide/2
  p,q,r/1 -> wxVb/1, J*w/1(p q r), wx(Jw)/1, "p,q,r "/1
  J*w/1("J*w ") -> wx(Jw)/2
  Constant2/1 -> vb/2
  f/1 -> a=f/m/1
  Product1/1 -> ve/1
  vb/1 -> wxVb/2, Product1/2, "vb "/1
  mass & inertia/1(m) -> a=f/m/2
  Rbe/1 -> Product1/1
  Reshape/1 -> p,q,r/1
  Constant1/1 -> p,q,r/2
  wxVb/1 -> Add/2
  Add/1 -> vb/1
  wx(Jw)/1 -> Add1/2, Scope1/2
  Mb/1 -> Add1/1, Scope1/1
  a=f/m/1 -> Add/1
  Constant4/1 -> mass & inertia/3(Jxx)
  Clock/1 -> mass & inertia/1(t)
  Constant5/1 -> mass & inertia/4(Jyy)
  Constant6/1 -> mass & inertia/5(Jzz)
  Constant3/1 -> mass & inertia/2("m ")

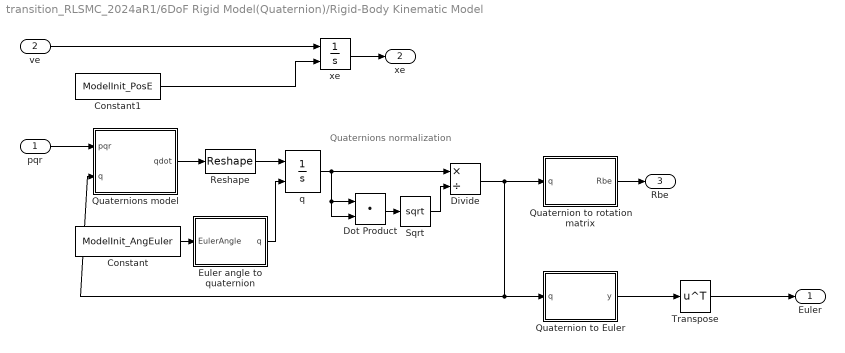
== system transition_RLSMC_2024aR1/6DoF Rigid Model(Quaternion)/Rigid-Body Kinematic Model  ==
  note: Quaternions
      | normalization
  pqr : Inport
  ve : Inport  Port=2
  Constant : Constant  Value=ModelInit_AngEuler
  Constant1 : Constant  Value=ModelInit_PosE
  Divide : Product  Inputs=*/
  Dot Product : DotProduct  OutDataTypeStr=Inherit: Inherit via internal rule
  Euler angle to quaternion : MATLAB Function
  Quaternion to Euler : MATLAB Function
  Quaternion to rotation matrix : MATLAB Function
  Quaternions model : MATLAB Function  TreatAsAtomicUnit=on
  Reshape : Reshape  OutputDimensionality=Customize  OutputDimensions=[4,1]
  Sqrt : Sqrt
  Transpose : Math  Operator=transpose
  q : Integrator  InitialConditionSource=external
  xe : Integrator  InitialConditionSource=external
  Euler : Outport  VectorParamsAs1DForOutWhenUnconnected=off
  "xe " : Outport  Port=2  VectorParamsAs1DForOutWhenUnconnected=off
  Rbe : Outport  Port=3  VectorParamsAs1DForOutWhenUnconnected=off
  wires:
  Divide/1 -> Quaternion to rotation matrix/1(q), Quaternions model/2(q), Quaternion to Euler/1(q)
  Dot Product/1 -> Sqrt/1
  pqr/1 -> Quaternions model/1(pqr)
  q/1 -> Divide/1, Dot Product/1, Dot Product/2
  Quaternions model/1(qdot) -> Reshape/1
  Quaternion to rotation matrix/1(Rbe) -> Rbe/1
  Quaternion to Euler/1(y) -> Transpose/1
  Constant/1 -> Euler angle to quaternion/1(EulerAngle)
  Euler angle to quaternion/1(q) -> q/2
  Reshape/1 -> q/1
  ve/1 -> xe/1
  xe/1 -> "xe "/1
  Constant1/1 -> xe/2
  Sqrt/1 -> Divide/2
  Transpose/1 -> Euler/1

== system transition_RLSMC_2024aR1/Control system/Signal Builder6 ==
  Demux : Demux  Tag=STV Demux  Outputs=1
      settings: DisplayOption=none
  FromWs : FromWorkspace  Tag=STV FromWs  VariableName=tuvar
      SigBuilderData=|
      | common.afterFinalStr = 'Extrapolate'
      | common.sampleTime = 0
      | dataSet.timeRange = [0 60]
      | dataSet.name = 'Group 1'
      | sbobj.Groups.Name = 'Group 1'
      | sbobj.Groups.Signals.Name = 'Signal 1'
      | sbobj.Groups.Signals.XData = [0 12.85 12.85 36.65 40 55.15 55.15 57.9 57.9 60]
      | sbobj.Groups.Signals.YData = [0 0 4 4 0 0 -4.1 -4.1 0 0]
      | sbobj.Groups.TimeRange = [0 60]
  Signal 1 : Outport  Tag=STV Outport
  wires:
  Demux/1 -> Signal 1/1
  FromWs/1 -> Demux/1

== system transition_RLSMC_2024aR1/Control system/Signal Builder7 ==
  Demux : Demux  Tag=STV Demux  Outputs=1
      settings: DisplayOption=none
  FromWs : FromWorkspace  Tag=STV FromWs  VariableName=tuvar
      SigBuilderData=|
      | common.afterFinalStr = 'Extrapolate'
      | common.sampleTime = 0
      | dataSet.timeRange = [0 60]
      | dataSet.name = 'Group 1'
      | sbobj.Groups.Name = 'Group 1'
      | sbobj.Groups.Signals.Name = 'Signal 1'
      | sbobj.Groups.Signals.XData = [0 11.9 11.9 24.2 24.2 28.2 28.2 38.8 38.8 60]
      | sbobj.Groups.Signals.YData = [0 0 -4.05 -4.05 0 0 4.05 4.05 0 0.00899587345254]
      | sbobj.Groups.TimeRange = [0 60]
  Signal 1 : Outport  Tag=STV Outport
  wires:
  Demux/1 -> Signal 1/1
  FromWs/1 -> Demux/1

== system transition_RLSMC_2024aR1/Control system/Single ==
  Demux : Demux  Tag=STV Demux  Outputs=1
      settings: DisplayOption=none
  FromWs : FromWorkspace  Tag=STV FromWs  VariableName=tuvar
      SigBuilderData=|
      | common.afterFinalStr = 'Extrapolate'
      | common.sampleTime = 0
      | dataSet.timeRange = [0 60]
      | dataSet.name = 'Group 1'
      | sbobj.Groups.Name = 'Group 1'
      | sbobj.Groups.Signals.Name = 'Signal 1'
      | sbobj.Groups.Signals.XData = [0 12 12 37.9 37.9 55.15 55.15 57.9 57.9 60]
      | sbobj.Groups.Signals.YData = [0 0 5 5 0 0 -4.1 -4.1 0 0]
      | sbobj.Groups.TimeRange = [0 60]
  Signal 1 : Outport  Tag=STV Outport
  wires:
  Demux/1 -> Signal 1/1
  FromWs/1 -> Demux/1

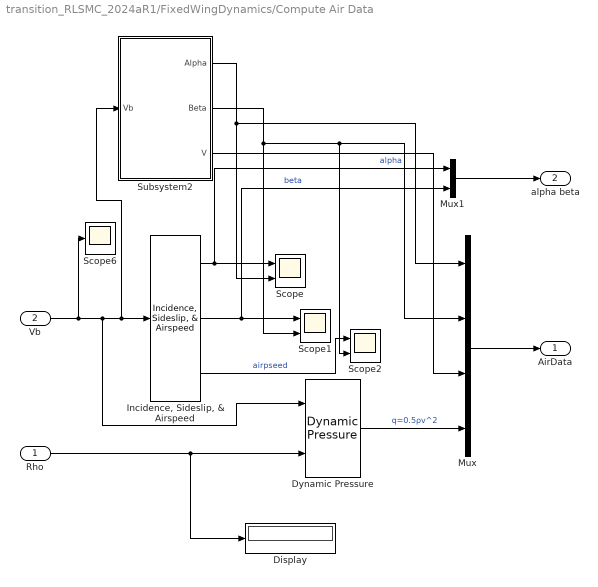
== system transition_RLSMC_2024aR1/FixedWingDynamics/Compute Air Data ==
  Rho : Inport
  Vb : Inport  Port=2  PortDimensions=3
  Display : Display
  Dynamic Pressure : aerolibasang/Dynamic Pressure
  "Incidence, Sideslip, & Airspeed" : aerolibasang/Incidence, Sideslip, & Airspeed
  Mux : Mux
  Mux1 : Mux  Inputs=2
  Scope : Scope  NumInputPorts=2
  Scope1 : Scope  NumInputPorts=2
  Scope2 : Scope  NumInputPorts=2
  Scope6 : Scope
  Subsystem2 : Subsystem
  AirData : Outport  VectorParamsAs1DForOutWhenUnconnected=off
  alpha beta : Outport  Port=2
  wires:
  Rho/1 -> Display/1, Dynamic Pressure/2
  Dynamic Pressure/1 -> Mux/4  "q=0.5ρv^2"
  Vb/1 -> Scope6/1, Subsystem2/1(Vb), "Incidence, Sideslip, & Airspeed"/1, Dynamic Pressure/1
  Mux/1 -> AirData/1
  Subsystem2/1(Alpha) -> Mux/1, Scope/2
  Subsystem2/2(Beta) -> Scope1/2, Scope2/2, Mux/2
  Subsystem2/3(V) -> Mux/3
  "Incidence, Sideslip, & Airspeed"/1 -> Mux1/1, Scope/1  "alpha"
  "Incidence, Sideslip, & Airspeed"/2 -> Mux1/2, Scope1/1  "beta"
  "Incidence, Sideslip, & Airspeed"/3 -> Scope2/1  "airpseed"
  Mux1/1 -> alpha beta/1

== system transition_RLSMC_2024aR1/FixedWingDynamics/Compute Rho ==
  note: Speed of Sound
  Xe : Inport
  COESA Atmosphere Model : aerolibatmos2/COESA Atmosphere Model  units=Metric (MKS)  spec=1976 COESA-extended U.S. Standard Atmosphere  model=Profile  profile_var=High temperature  profile_percent=10%  profile_alt=5 km (16404 ft)  envelope_var=High temperature  envelope_percent=1%  action=None
  Get Z : Selector  InputPortWidth=3  IndexOptions=Index vector (dialog)  Indices=[3]  OutputSizes=[(-2)]
  Terminator3 : Terminator
  Terminator4 : Terminator
  Terminator6 : Terminator
  z-->h : Abs
  Rho : Outport  VectorParamsAs1DForOutWhenUnconnected=off
  wires:
  Xe/1 -> Get Z/1
  Get Z/1 -> z-->h/1
  COESA Atmosphere Model/2 -> Terminator6/1
  COESA Atmosphere Model/4 -> Rho/1
  COESA Atmosphere Model/1 -> Terminator3/1
  COESA Atmosphere Model/3 -> Terminator4/1
  z-->h/1 -> COESA Atmosphere Model/1

== system transition_RLSMC_2024aR1/FixedWingDynamics/Rotate FM to body frame ==
  FM_w : Inport
  alpha_beta : Inport  Port=2
  Forces : Selector  InputPortWidth=6  IndexOptions=Index vector (dialog)  Indices=[1 2 3]  OutputSizes=[(-2)]
  Moments : Selector  InputPortWidth=6  IndexOptions=Index vector (dialog)  Indices=[4 5 6]  OutputSizes=[(-2)]
  Rotate Forces : Subsystem
  F_b : Outport  VectorParamsAs1DForOutWhenUnconnected=off
  M_b : Outport  Port=2  VectorParamsAs1DForOutWhenUnconnected=off
  wires:
  alpha_beta/1 -> Rotate Forces/2(alpha_beta)
  FM_w/1 -> Forces/1, Moments/1
  Forces/1 -> Rotate Forces/1(F_w)
  Rotate Forces/1(F_b) -> F_b/1
  Moments/1 -> M_b/1

== system transition_RLSMC_2024aR1/FixedWingDynamics/Rotate Vw ==
  Vw : Inport
  Euler : Inport  Port=2
  RL2B : Subsystem
  RL2B * Vw : Product  Multiplication=Matrix(*)  InputSameDT=on  SaturateOnIntegerOverflow=on  OutDataTypeStr=Inherit: Same as first input
  Vb : Outport  Unit=m/s  VectorParamsAs1DForOutWhenUnconnected=off
  wires:
  RL2B * Vw/1 -> Vb/1
  Vw/1 -> RL2B * Vw/2
  RL2B/1(RL2B) -> RL2B * Vw/1
  Euler/1 -> RL2B/1(Euler)

== system transition_RLSMC_2024aR1/Gravity (To Body Frame)/Rotate g to Body Frame ==
  Euler : Inport
  Gravity Force : Inport  Port=2  PortDimensions=3
  Product1 : Product  Multiplication=Matrix(*)  InputSameDT=on  SaturateOnIntegerOverflow=on  OutDataTypeStr=Inherit: Same as first input
  RL2B : Subsystem
  g_b : Outport  Unit=kg*m/s^2  VectorParamsAs1DForOutWhenUnconnected=off
  wires:
  Gravity Force/1 -> Product1/2
  Euler/1 -> RL2B/1(Euler)
  Product1/1 -> g_b/1
  RL2B/1(RL2B) -> Product1/1

== system transition_RLSMC_2024aR1/6DoF Rigid Model(Quaternion)/Rigid-Body Dynamic Model/J*w ==
  p q r : Inport
  J : Inport  Port=2
  J*w : Product  Multiplication=Matrix(*)
  "J*w " : Outport  VectorParamsAs1DForOutWhenUnconnected=off
  wires:
  J*w/1 -> "J*w "/1
  J/1 -> J*w/1
  p q r/1 -> J*w/2

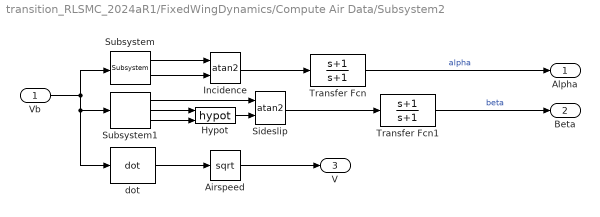
== system transition_RLSMC_2024aR1/FixedWingDynamics/Compute Air Data/Subsystem2 ==
  Vb : Inport
  Airspeed : Sqrt  AlgorithmType=Newton-Raphson
  Hypot : Math  Operator=hypot
  Incidence : Trigonometry  Operator=atan2
  Sideslip : Trigonometry  Operator=atan2
  Subsystem : aerolibasang/Incidence, Sideslip, & Airspeed/Subsystem  SystemSampleTime=-1  VariantActivationTime=update diagram  AllowFlexibleInterface=on  Latency=0  AutoFrameSizeCalculation=off
  Subsystem1 : aerolibasang/Incidence, Sideslip, & Airspeed/Subsystem1  SystemSampleTime=-1  VariantActivationTime=update diagram  AllowFlexibleInterface=on  Latency=0  AutoFrameSizeCalculation=off
  Transfer Fcn : TransferFcn  Numerator=[1 1]  Denominator=[1 1]
  Transfer Fcn1 : TransferFcn  Numerator=[1 1]  Denominator=[1 1]
  dot : aerolibasang/Incidence, Sideslip, & Airspeed/dot  SystemSampleTime=-1  VariantActivationTime=update diagram  AllowFlexibleInterface=on  Latency=0  AutoFrameSizeCalculation=off
  Alpha : Outport  Unit=rad  InitialOutput=0  VectorParamsAs1DForOutWhenUnconnected=off
  Beta : Outport  Port=2  Unit=rad  InitialOutput=0  VectorParamsAs1DForOutWhenUnconnected=off
  V : Outport  Port=3  InitialOutput=0  VectorParamsAs1DForOutWhenUnconnected=off
  wires:
  Subsystem/2 -> Incidence/2
  dot/1 -> Airspeed/1
  Vb/1 -> Subsystem/1, Subsystem1/1, dot/1
  Incidence/1 -> Transfer Fcn/1
  Subsystem1/3 -> Hypot/2
  Hypot/1 -> Sideslip/2
  Subsystem1/1 -> Sideslip/1
  Sideslip/1 -> Transfer Fcn1/1
  Airspeed/1 -> V/1
  Subsystem1/2 -> Hypot/1
  Subsystem/1 -> Incidence/1
  Transfer Fcn/1 -> Alpha/1  "alpha"
  Transfer Fcn1/1 -> Beta/1  "beta"

== system transition_RLSMC_2024aR1/FixedWingDynamics/Rotate FM to body frame/Rotate Forces ==
  F_w : Inport
  alpha_beta : Inport  Port=2
  Product2 : Product  Multiplication=Matrix(*)  SaturateOnIntegerOverflow=on  OutDataTypeStr=Inherit: Same as first input
  RB2W : Subsystem
  RW2B : Math  Operator=transpose  SignedPower=on
  F_b : Outport  PortDimensions=3  VectorParamsAs1DForOutWhenUnconnected=off
  wires:
  RW2B/1 -> Product2/1
  F_w/1 -> Product2/2
  Product2/1 -> F_b/1
  alpha_beta/1 -> RB2W/1(aoa beta)
  RB2W/1(Rw2b) -> RW2B/1

== system transition_RLSMC_2024aR1/FixedWingDynamics/Rotate Vw/RL2B ==
  Euler : Inport
  Rotation Angles to Direction Cosine Matrix : sharedtransform/Rotation Angles to Direction Cosine Matrix  rotationOrder=ZYX  aMode=aMode
  Selector : Selector  InputPortWidth=3  IndexOptions=Index vector (dialog)  Indices=[3 2 1]  OutputSizes=1
  RL2B : Outport  VectorParamsAs1DForOutWhenUnconnected=off
  wires:
  Rotation Angles to Direction Cosine Matrix/1 -> RL2B/1
  Euler/1 -> Selector/1
  Selector/1 -> Rotation Angles to Direction Cosine Matrix/1

== system transition_RLSMC_2024aR1/Gravity (To Body Frame)/Rotate g to Body Frame/RL2B ==
  Euler : Inport
  Rotation Angles to Direction Cosine Matrix : sharedtransform/Rotation Angles to Direction Cosine Matrix  rotationOrder=ZYX  aMode=aMode
  Selector : Selector  InputPortWidth=3  IndexOptions=Index vector (dialog)  Indices=[3 2 1]  OutputSizes=1
  RL2B : Outport  VectorParamsAs1DForOutWhenUnconnected=off
  wires:
  Rotation Angles to Direction Cosine Matrix/1 -> RL2B/1
  Euler/1 -> Selector/1
  Selector/1 -> Rotation Angles to Direction Cosine Matrix/1

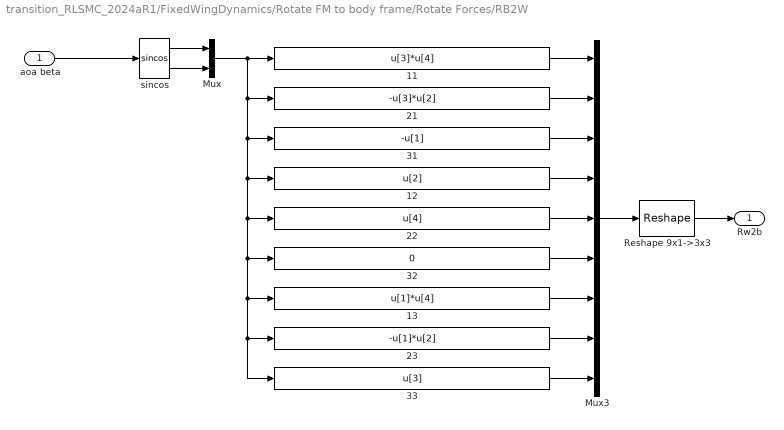
== system transition_RLSMC_2024aR1/FixedWingDynamics/Rotate FM to body frame/Rotate Forces/RB2W ==
  aoa beta : Inport
  11 : Fcn  Expr=u[3]*u[4]
  12 : Fcn  Expr=u[2]
  13 : Fcn  Expr=u[1]*u[4]
  21 : Fcn  Expr=-u[3]*u[2]
  22 : Fcn  Expr=u[4]
  23 : Fcn  Expr=-u[1]*u[2]
  31 : Fcn  Expr=-u[1]
  32 : Fcn  Expr=0
  33 : Fcn  Expr=u[3]
  Mux : Mux  Inputs=2
  Mux3 : Mux  Inputs=9
  Reshape 9x1->3x3 : Reshape  OutputDimensionality=Customize  OutputDimensions=[3,3]
  sincos : Trigonometry  Operator=sincos
  Rw2b : Outport  VectorParamsAs1DForOutWhenUnconnected=off
  wires:
  Mux/1 -> 11/1, 21/1, 31/1, 12/1, 22/1, 32/1, 13/1, 23/1, 33/1
  aoa beta/1 -> sincos/1
  sincos/2 -> Mux/2
  sincos/1 -> Mux/1
  33/1 -> Mux3/9
  23/1 -> Mux3/8
  13/1 -> Mux3/7
  32/1 -> Mux3/6
  22/1 -> Mux3/5
  12/1 -> Mux3/4
  31/1 -> Mux3/3
  21/1 -> Mux3/2
  11/1 -> Mux3/1
  Reshape 9x1->3x3/1 -> Rw2b/1
  Mux3/1 -> Reshape 9x1->3x3/1

== matlab function transition_RLSMC_2024aR1/QuadcoptersDynamics/Quadcopters Force & Moment ==
  data: Fb_cm output; Kf input; Kt input; Lr input; Mb_cm output; Lp input; g input; Izz input
function [Fb_cm,Mb_cm] = fcn(Kf,Kt,Lr,Lp,g,Izz)

Fb_cm = [Kf*g,Kf*g,Kf*g,Kf*g];
Mb_cm = [-Lr*Kf*g            Lr*Kf*g             Lr*Kf*g           -Lr*Kf*g
          Lp*Kf*g           -Lp*Kf*g             Lp*Kf*g           -Lp*Kf*g
          Kt*Izz            Kt*Izz              -Kt*Izz            -Kt*Izz              ];

== matlab function transition_RLSMC_2024aR1/6DoF Rigid Model(Quaternion)/Rigid-Body Kinematic Model /Euler angle to quaternion ==
  data: EulerAngle input; q output
function q = fcn(EulerAngle)
%Function description:
%  Get quaternions from Euler angle
q0 =  cos(EulerAngle(1)/2)*cos(EulerAngle(2)/2)*cos(EulerAngle(3)/2) + sin(EulerAngle(1)/2)*sin((EulerAngle(2)/2))*sin((EulerAngle(3)/2));
q1 = sin(EulerAngle(1)/2)*cos(EulerAngle(2)/2)*cos(EulerAngle(3)/2) - cos(EulerAngle(1)/2)*sin((EulerAngle(2)/2))*sin((EulerAngle(3)/2));
q2 = cos(EulerAngle(1)/2)*sin(EulerAngle(2)/2)*cos(EulerAngle(3)/2) + sin(EulerAngle(1)/2)*cos((EulerAngle(2)/2))*sin((EulerAngle(3)/2));
q3 = cos(EulerAngle(1)/2)*cos(EulerAngle(2)/2)*sin(EulerAngle(3)/2) - sin(EulerAngle(1)/2)*sin((EulerAngle(2)/2))*cos((EulerAngle(3)/2));
q = [q0 q1 q2 q3]';

== matlab function transition_RLSMC_2024aR1/6DoF Rigid Model(Quaternion)/Rigid-Body Kinematic Model /Quaternion to Euler ==
  data: q input; y output
function y = fcn(q)
 %Function description:
%  Quaternions to Euler
phi = atan2(2*(q(1)*q(2) + q(3)*q(4)), (1 - 2*(q(2)*q(2) + q(3)*q(3))));
theta = asin(2*(q(1)*q(3) - q(2)*q(4)));
psi = atan2(2*(q(1)*q(4) + q(2)*q(3)), (1 - 2*(q(3)*q(3) + q(4)*q(4))));
y = [phi theta psi];

== matlab function transition_RLSMC_2024aR1/6DoF Rigid Model(Quaternion)/Rigid-Body Kinematic Model /Quaternion to rotation matrix ==
  data: q input; Rbe output
function Rbe = fcn(q)
%Function description;
%  The rotation matrix of the Aircraft-Body Coordinate Frame (ABCF) to the
%  Earth-Fixed Coordinate Frame (EFCF) is obtained from the quaternions
Rbe = [q(1)*q(1) + q(2)*q(2) - q(3)*q(3) - q(4)*q(4), 2*(q(2)*q(3) - q(1)*q(4)), 2*(q(2)*q(4) + q(1)*q(3))
           2*(q(2)*q(3) + q(1)*q(4)), q(1)*q(1) - q(2)*q(2) + q(3)*q(3) - q(4)*q(4), 2*(q(3)*q(4) - q(1)*q(2))
           2*(q(2)*q(4) - q(1)*q(3)), 2*(q(3)*q(4) + q(1)*q(2)), q(1)*q(1) - q(2)*q(2) - q(3)*q(3) + q(4)*q(4)];

== matlab function transition_RLSMC_2024aR1/6DoF Rigid Model(Quaternion)/Rigid-Body Kinematic Model /Quaternions model ==
  data: pqr input; qdot output; q input
function qdot = fcn(pqr, q)
%Function description:
%  Quaternions model
qdot = 0.5*[0, -pqr(1), -pqr(2), -pqr(3); pqr(1), 0, pqr(3), -pqr(2); pqr(2), -pqr(3), 0, pqr(1); pqr(3), pqr(2), -pqr(1), 0]*q;

== matlab function transition_RLSMC_2024aR1/6DoF Rigid Model(Quaternion)/Rigid-Body Dynamic Model/mass & inertia ==
  data: t input; m output; J output; m input; Jxx input; Jyy input; Jzz input
function [m,J] = fcn(t,m,Jxx,Jyy,Jzz)

if t<60
    m = m;
else
    m = 0.8*m;
end
% m = m+5*sin(pi*t);
% if t<15
%     Jxx = Jxx;
%     Jyy = Jyy;
%     Jzz = Jzz;
% else
%     Jxx = 0.8*Jxx;
%     Jyy = 0.8*Jyy;
%     Jzz = 0.8*Jzz;
% end

% m = m;

J = diag([Jxx,Jyy,Jzz]);

end
